simulink model "sldemo_lct_fixpt_params"  (Simulink 7.6)
settings: Solver=FixedStepDiscrete  StartTime=0.0  StopTime=10.0  FixedStep=0.1  RelTol=1e-3
PreLoadFcn:
  | load sldemo_lct_data.mat
  | 
  | Kinline = 2;
  | 
  | Kcs = 2;
  | 
  | KmyFixpt = Simulink.Parameter;
  | KmyFixpt.Value = 2;
  | KmyFixpt.DataType = 'myFixpt';
  | KmyFixpt.RTWInfo.StorageClass = 'ExportedGlobal';
  | 
  | Kuint8 = Simulink.Parameter;
  | Kuint8.Value = 2;
  | Kuint8.DataType = 'uint8';
  | Kuint8.RTWInfo.StorageClass = 'ExportedGlobal';
undefined symbols (not defined in the file or in its folder): myFixpt
Description:
  | Fixed Point Parameters
settings Model: MinMaxOverflowLogging=MinMaxAndOverflow  Creator=The MathWorks Inc.  ExtModeAutoUpdateStatusClock=off  TunableVars=Kcs  TunableVarsStorageClass=ExportedGlobal
settings DataIOCC: SaveOutput=off  SaveTime=off  SignalLoggingName=logsOut
settings OptimizationCC: InlineParams=on  InlineInvariantSignals=on  ZeroExternalMemoryAtStartup=off  ZeroInternalMemoryAtStartup=off  InitFltsAndDblsToZero=on  NoFixptDivByZeroProtection=on  EfficientFloat2IntCast=on  OptimizeModelRefInitCode=on  LifeSpan=1
settings DebuggingCC: SaveWithParameterizedLinksMsg=none  SignalResolutionControl=TryResolveAllWithWarning  SolverPrmCheckMsg=none  MultiTaskDSMMsg=warning  MultiTaskCondExecSysMsg=none
settings HardwareCC: TargetUnknown=on
settings RTWCC: SystemTargetFile=ert.tlc  TemplateMakefile=ert_default_tmf  Description=RTW Embedded Coder (no auto configuration)  GenerateReport=on  ProcessScript=ert_make_rtw_hook  IncludeHyperlinkInReport=on  LaunchReport=on  IncludeERTFirstTime=on
settings CodeAppCC: IgnoreCustomStorageClasses=off
settings ERTTargetCC: TargetFcnLib=ansi_tfl_tmw.mat  MultiwordLength=2048  GenerateSampleERTMain=on  IncludeMdlTerminateFcn=off  SuppressErrorStatus=on  SupportAbsoluteTime=off  SupportNonFinite=off  SupportComplex=off  InlinedParameterPlacement=NonHierarchical  ERTSrcFileBannerTemplate=example_banner.tlc  ERTHdrFileBannerTemplate=example_banner.tlc  ERTCustomFileTemplate=example_file_process.tlc  ConvertIfToSwitch=off

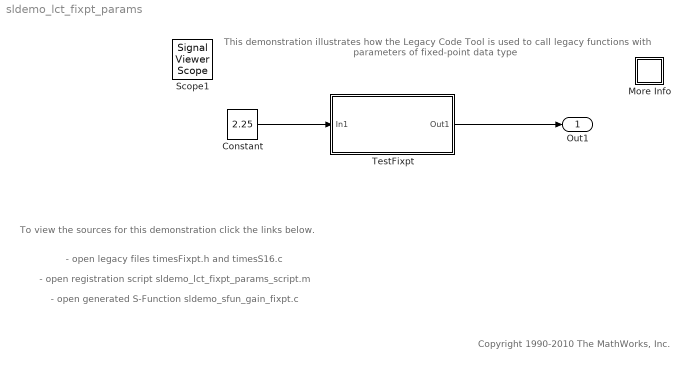
== system sldemo_lct_fixpt_params ==
  note: Copyright 1990-2010 The MathWorks, Inc.
  note: This demonstration illustrates how the Legacy Code Tool is used to
      | call legacy functions with parameters of fixed-point data type
  note: - open legacy files timesFixpt.h and timesS16.c
  note: To view the sources for this demonstration
      | click the links below.
  note: - open registration script sldemo_lct_fixpt_params_script.m
  note: - open generated S-Function sldemo_sfun_gain_fixpt.c
  Constant : Constant  Value=2.25  OutDataTypeStr=myFixpt  SampleTime=0.1
  More Info : Subsystem
      settings: OpenFcn=showdemo('sldemo_lct_fixpt_params_script')
      mask Display: disp('?')
  TestFixpt : Subsystem
  Out1 : Outport
  Scope1 : SignalViewerScope  IOType=viewer  RefreshTime=0.035000
  wires:
  Constant/1 -> TestFixpt/1(In1)
  TestFixpt/1(Out1) -> Out1/1

== system sldemo_lct_fixpt_params/More Info ==

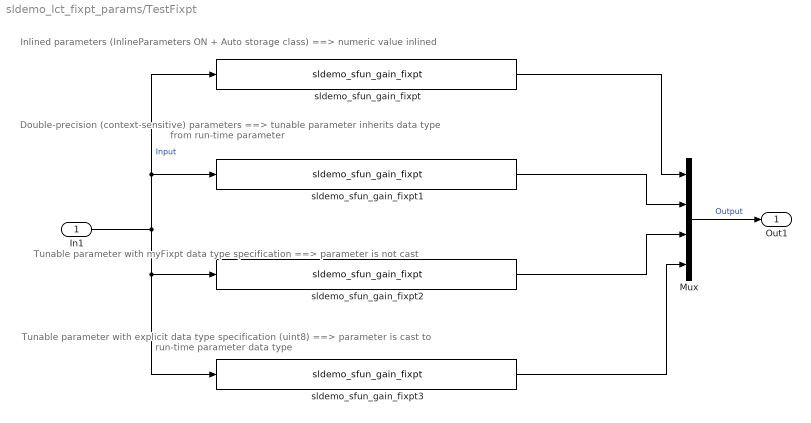
== system sldemo_lct_fixpt_params/TestFixpt ==
  note: Inlined parameters (InlineParameters ON + Auto storage class)
      | ==> numeric value inlined
  note: Tunable parameter with myFixpt data type specification
      | ==> parameter is not cast
  note: Double-precision (context-sensitive) parameters
      | ==> tunable parameter inherits data type from run-time parameter
  note: Tunable parameter with explicit data type specification (uint8)
      | ==> parameter is cast to run-time parameter data type
  In1 : Inport  OutDataTypeStr=myFixpt
  Mux : Mux
  sldemo_sfun_gain_fixpt : S-Function  FunctionName=sldemo_sfun_gain_fixpt  Parameters=SParameter1, SParameter2  EnableBusSupport=off  mask(Legacy Function){SFunctionSpec=myFixpt y1 = timesS16(myFixpt u1, myFixpt p1, uint8 p2), SParameter1=Kinline, SParameter2=myFixpt.FractionLength, ShowSpec=on}
      mask prompts: SParameter1 "P1:"; SParameter2 "P2:"; ShowSpec "Display function specification"
      mask help:
      | This block allows you to call the legacy functions specified by the following Legacy Code Tool definition:
      | def.SFunctionName = 'sldemo_sfun_gain_fixpt';
      | def.OutputFcnSpec = 'myFixpt y1 = timesS16(myFixpt u1, myFixpt p1, uint8 p2)';
      | def.HeaderFiles = {'timesFixpt.h'};
      | def.SourceFiles = {'timesS16.c'};
      | def.IncPaths = {'sldemo_lct_src'};
      | def.SrcPaths = {'sldemo_lct_src'};
      mask Help: <p>This block was generated automatically by the Legacy Code Tool. For detailed help on this tool, call<a href="matlab:legacy_code('help')"> legacy_code('help')</a>.</p>
      mask CallbackString:
      | |||if strcmp(get_param(gcbh, 'ShowSpec'), 'on')
      |   set_param(gcbh, 'MaskDisplay', sprintf('fprintf(''%s'');', get_param(gcbh, 'SFunctionSpec')));
      | else
      |   set_param(gcbh, 'MaskDisplay', sprintf('fprintf(''%s'');', get_param(gcbh, 'FunctionName')));
      | end
      mask Display: fprintf('myFixpt y1 = timesS16(myFixpt u1, myFixpt p1, uint8 p2)');
  sldemo_sfun_gain_fixpt1 : S-Function  FunctionName=sldemo_sfun_gain_fixpt  Parameters=SParameter1, SParameter2  EnableBusSupport=off  mask(Legacy Function){SFunctionSpec=myFixpt y1 = timesS16(myFixpt u1, myFixpt p1, uint8 p2), SParameter1=Kcs, SParameter2=myFixpt.FractionLength, ShowSpec=on}
      mask prompts: SParameter1 "P1:"; SParameter2 "P2:"; ShowSpec "Display function specification"
      mask help:
      | This block allows you to call the legacy functions specified by the following Legacy Code Tool definition:
      | def.SFunctionName = 'sldemo_sfun_gain_fixpt';
      | def.OutputFcnSpec = 'myFixpt y1 = timesS16(myFixpt u1, myFixpt p1, uint8 p2)';
      | def.HeaderFiles = {'timesFixpt.h'};
      | def.SourceFiles = {'timesS16.c'};
      | def.IncPaths = {'sldemo_lct_src'};
      | def.SrcPaths = {'sldemo_lct_src'};
      mask Help: <p>This block was generated automatically by the Legacy Code Tool. For detailed help on this tool, call<a href="matlab:legacy_code('help')"> legacy_code('help')</a>.</p>
      mask CallbackString:
      | |||if strcmp(get_param(gcbh, 'ShowSpec'), 'on')
      |   set_param(gcbh, 'MaskDisplay', sprintf('fprintf(''%s'');', get_param(gcbh, 'SFunctionSpec')));
      | else
      |   set_param(gcbh, 'MaskDisplay', sprintf('fprintf(''%s'');', get_param(gcbh, 'FunctionName')));
      | end
      mask Display: fprintf('myFixpt y1 = timesS16(myFixpt u1, myFixpt p1, uint8 p2)');
  sldemo_sfun_gain_fixpt2 : S-Function  FunctionName=sldemo_sfun_gain_fixpt  Parameters=SParameter1, SParameter2  EnableBusSupport=off  mask(Legacy Function){SFunctionSpec=myFixpt y1 = timesS16(myFixpt u1, myFixpt p1, uint8 p2), SParameter1=KmyFixpt, SParameter2=myFixpt.FractionLength, ShowSpec=on}
      mask prompts: SParameter1 "P1:"; SParameter2 "P2:"; ShowSpec "Display function specification"
      mask help:
      | This block allows you to call the legacy functions specified by the following Legacy Code Tool definition:
      | def.SFunctionName = 'sldemo_sfun_gain_fixpt';
      | def.OutputFcnSpec = 'myFixpt y1 = timesS16(myFixpt u1, myFixpt p1, uint8 p2)';
      | def.HeaderFiles = {'timesFixpt.h'};
      | def.SourceFiles = {'timesS16.c'};
      | def.IncPaths = {'sldemo_lct_src'};
      | def.SrcPaths = {'sldemo_lct_src'};
      mask Help: <p>This block was generated automatically by the Legacy Code Tool. For detailed help on this tool, call<a href="matlab:legacy_code('help')"> legacy_code('help')</a>.</p>
      mask CallbackString:
      | |||if strcmp(get_param(gcbh, 'ShowSpec'), 'on')
      |   set_param(gcbh, 'MaskDisplay', sprintf('fprintf(''%s'');', get_param(gcbh, 'SFunctionSpec')));
      | else
      |   set_param(gcbh, 'MaskDisplay', sprintf('fprintf(''%s'');', get_param(gcbh, 'FunctionName')));
      | end
      mask Display: fprintf('myFixpt y1 = timesS16(myFixpt u1, myFixpt p1, uint8 p2)');
  sldemo_sfun_gain_fixpt3 : S-Function  FunctionName=sldemo_sfun_gain_fixpt  Parameters=SParameter1, SParameter2  EnableBusSupport=off  mask(Legacy Function){SFunctionSpec=myFixpt y1 = timesS16(myFixpt u1, myFixpt p1, uint8 p2), SParameter1=Kuint8, SParameter2=myFixpt.FractionLength, ShowSpec=on}
      mask prompts: SParameter1 "P1:"; SParameter2 "P2:"; ShowSpec "Display function specification"
      mask help:
      | This block allows you to call the legacy functions specified by the following Legacy Code Tool definition:
      | def.SFunctionName = 'sldemo_sfun_gain_fixpt';
      | def.OutputFcnSpec = 'myFixpt y1 = timesS16(myFixpt u1, myFixpt p1, uint8 p2)';
      | def.HeaderFiles = {'timesFixpt.h'};
      | def.SourceFiles = {'timesS16.c'};
      | def.IncPaths = {'sldemo_lct_src'};
      | def.SrcPaths = {'sldemo_lct_src'};
      mask Help: <p>This block was generated automatically by the Legacy Code Tool. For detailed help on this tool, call<a href="matlab:legacy_code('help')"> legacy_code('help')</a>.</p>
      mask CallbackString:
      | |||if strcmp(get_param(gcbh, 'ShowSpec'), 'on')
      |   set_param(gcbh, 'MaskDisplay', sprintf('fprintf(''%s'');', get_param(gcbh, 'SFunctionSpec')));
      | else
      |   set_param(gcbh, 'MaskDisplay', sprintf('fprintf(''%s'');', get_param(gcbh, 'FunctionName')));
      | end
      mask Display: fprintf('myFixpt y1 = timesS16(myFixpt u1, myFixpt p1, uint8 p2)');
  Out1 : Outport
  wires:
  In1/1 -> sldemo_sfun_gain_fixpt2/1, sldemo_sfun_gain_fixpt3/1, sldemo_sfun_gain_fixpt1/1, sldemo_sfun_gain_fixpt/1  "Input"
  Mux/1 -> Out1/1  "Output"
  sldemo_sfun_gain_fixpt/1 -> Mux/1
  sldemo_sfun_gain_fixpt3/1 -> Mux/4
  sldemo_sfun_gain_fixpt1/1 -> Mux/2
  sldemo_sfun_gain_fixpt2/1 -> Mux/3
